simulink model "Q3_A"  (R2021b)
settings: Solver=VariableStepAuto  StartTime=0.0  StopTime=10  RelTol=1e-3
settings Model: Creator=alimi  LastModifiedBy=alimi

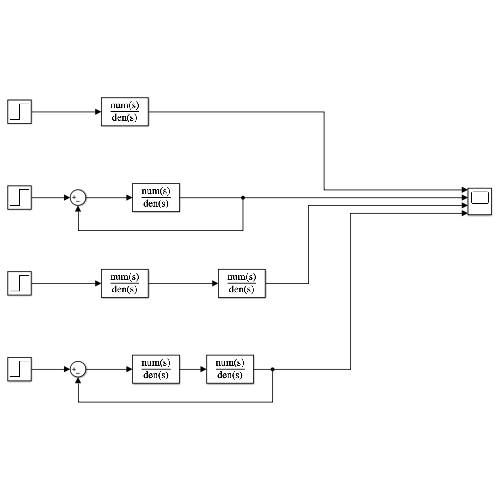
[thumbnail: Simulink's stored preview of the top-level diagram]
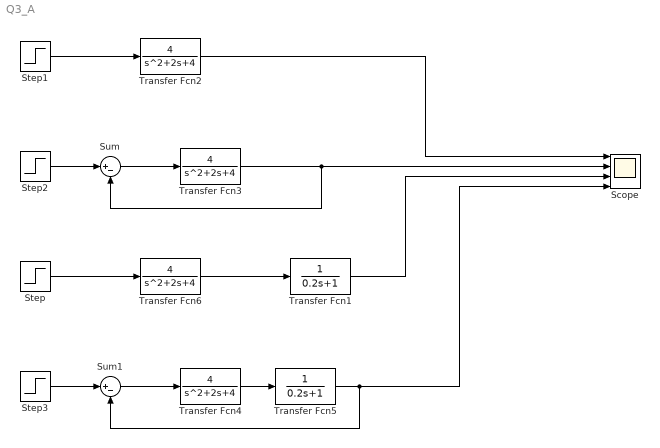
== system Q3_A ==
  Scope : Scope  NumInputPorts=4
  Step{,1..3} (4 alike) : Step  Time=0.001  SampleTime=0
  Sum : Sum  Inputs=|+-
  Sum1 : Sum  Inputs=|+-
  Transfer Fcn1 : TransferFcn  Denominator=[0.2 1]
  Transfer Fcn{2..4,6} (4 alike) : TransferFcn  Numerator=[4]  Denominator=[1 2 4]
  Transfer Fcn5 : TransferFcn  Denominator=[0.2 1]
  wires:
  Step/1 -> Transfer Fcn6/1
  Transfer Fcn6/1 -> Transfer Fcn1/1
  Step1/1 -> Transfer Fcn2/1
  Transfer Fcn2/1 -> Scope/1
  Step2/1 -> Sum/1
  Sum/1 -> Transfer Fcn3/1
  Transfer Fcn3/1 -> Sum/2, Scope/2
  Sum1/1 -> Transfer Fcn4/1
  Transfer Fcn4/1 -> Transfer Fcn5/1
  Transfer Fcn5/1 -> Scope/4, Sum1/2
  Step3/1 -> Sum1/1
  Transfer Fcn1/1 -> Scope/3
